simulink model "PWM"  (R2021a)
settings: Solver=VariableStepDiscrete  StartTime=0.0  StopTime=0.4  MaxStep=0.001  RelTol=1e-3
libraries: simulink x1, spspowerguiLib x1
settings Model: Creator=SA  LastModifiedBy=SA

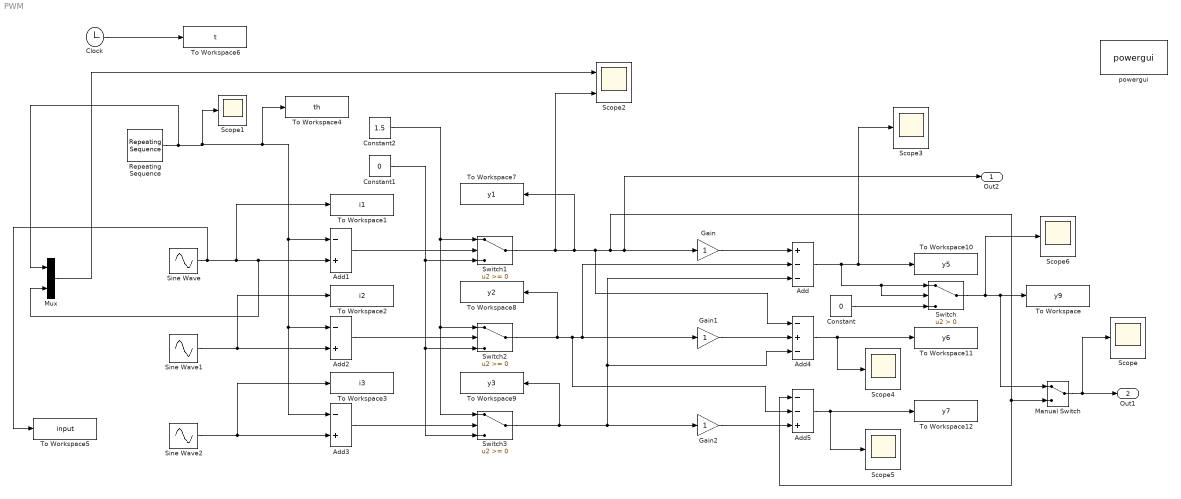
== system PWM ==
  Add : Sum  Inputs=+--
  Add1 : Sum  Inputs=-+
  Add2 : Sum  Inputs=-+
  Add3 : Sum  Inputs=-+
  Add4 : Sum  Inputs=-+-
  Add5 : Sum  Inputs=--+
  Clock : Clock
  Constant : Constant  Value=0
  Constant1 : Constant  Value=0
  Constant2 : Constant  Value=1.5
  Gain : Gain
  Gain1 : Gain
  Gain2 : Gain
  Manual Switch : ManualSwitch
  Mux : Mux  Inputs=2
  Repeating Sequence : simulink/Sources/Repeating Sequence  rep_seq_t=[0 0.1]  rep_seq_y=[0 0.9]
  Scope{,1,3..6} (6 alike) : Scope
  Scope2 : Scope  NumInputPorts=2
  Sine Wave : Sin  Frequency=60  SampleTime=0
  Sine Wave1 : Sin  Frequency=60  Phase=120  SampleTime=0
  Sine Wave2 : Sin  Frequency=60  Phase=-120  SampleTime=0
  Switch : Switch  Criteria=u2 > Threshold
  Switch1 : Switch
  Switch2 : Switch
  Switch3 : Switch
  To Workspace : ToWorkspace  VariableName=y9  SaveFormat=Timeseries  SampleTime=-1
  To Workspace1 : ToWorkspace  VariableName=i1  SaveFormat=Timeseries  SampleTime=-1
  To Workspace10 : ToWorkspace  VariableName=y5  SaveFormat=Timeseries  SampleTime=-1
  To Workspace11 : ToWorkspace  VariableName=y6  SaveFormat=Timeseries  SampleTime=-1
  To Workspace12 : ToWorkspace  VariableName=y7  SaveFormat=Timeseries  SampleTime=-1
  To Workspace2 : ToWorkspace  VariableName=i2  SaveFormat=Timeseries  SampleTime=-1
  To Workspace3 : ToWorkspace  VariableName=i3  SaveFormat=Timeseries  SampleTime=-1
  To Workspace4 : ToWorkspace  VariableName=th  SaveFormat=Timeseries  SampleTime=-1
  To Workspace5 : ToWorkspace  VariableName=input  SaveFormat=Timeseries  SampleTime=-1
  To Workspace6 : ToWorkspace  VariableName=t  SaveFormat=Timeseries  SampleTime=-1
  To Workspace7 : ToWorkspace  VariableName=y1  SaveFormat=Timeseries  SampleTime=-1
  To Workspace8 : ToWorkspace  VariableName=y2  SaveFormat=Timeseries  SampleTime=-1
  To Workspace9 : ToWorkspace  VariableName=y3  SaveFormat=Timeseries  SampleTime=-1
  powergui : spspowerguiLib/powergui  Priority=1  SimulationMode=Discrete  SampleTime=5e-5  frequency=60  Iterations=50  frequencyindice=60  Pbase=100e6  ErrMax=1e-4  UnitsV=kV  UnitsW=MW  buscounter=0  FunctionMessages=off  echomessages=off  EnableUseOfTLC=off  CurrentSourceSwitches=off  DisableSnubberDevices=off  DisableRonSwitches=off  DisableVfSwitches=off  DisplayEquations=off  AutomaticDiscreteSolvers=off  SolverType=Tustin/Backward Euler (TBE)  Interpol=off  ExternalGateDelay=off  methode=off  Ts=100  x0status=blocks  SPID=on  SwTol=0  HookPort=off  NonlinearTolerance=1e-4  nMaxIteration=100  ContinueOnMaxIteration=off  RestoreLinks=warning  ResistiveCurrentMeasurement=off  Frange=[0:2:500]  Ylog=off  Xlog=on  ShowGrid=off  save=off  variable=ZData  structure=0  ZoomFFT=off  StartTime=0.0  cycles=1  DisplayStyle=1  fundamental=60  FreqAxis=off  MaxFrequency=1000  frequencyindicesteady=1  RmsSteady=1  display=off
  Out2 : Outport
  Out1 : Outport  Port=2
  wires:
  Sine Wave/1 -> To Workspace5/1, Add1/2, Mux/2, To Workspace1/1
  Sine Wave1/1 -> Add2/2, To Workspace2/1
  Sine Wave2/1 -> Add3/2, To Workspace3/1
  Repeating Sequence/1 -> Mux/1, Add2/1, Add3/1, Add1/1, To Workspace4/1, Scope1/1
  Clock/1 -> To Workspace6/1
  Mux/1 -> Scope2/1
  Add1/1 -> Switch1/2
  Add2/1 -> Switch2/2
  Add3/1 -> Switch3/2
  Constant1/1 -> Switch1/3, Switch2/3, Switch3/3
  Constant2/1 -> Switch3/1, Switch2/1, Switch1/1
  Gain/1 -> Add/1
  Gain1/1 -> Add4/2
  Gain2/1 -> Add5/3
  Switch1/1 -> Scope2/2, Add4/1, Add5/1, Manual Switch/2, Out2/1, Gain/1, To Workspace7/1
  Switch2/1 -> To Workspace8/1, Add/2, Gain1/1, Add5/2
  Switch3/1 -> To Workspace9/1, Add/3, Add4/3, Gain2/1
  Constant/1 -> Switch/3
  Add/1 -> To Workspace10/1, Scope3/1, Switch/2, Switch/1
  Add4/1 -> Scope4/1, To Workspace11/1
  Add5/1 -> Scope5/1, To Workspace12/1
  Switch/1 -> Scope6/1, Manual Switch/1, To Workspace/1
  Manual Switch/1 -> Scope/1, Out1/1
